simulink model "GMCLIB_Clark_BAM_FLT"  (Simulink 7.3)
settings: Solver=ode45  StartTime=0.0  StopTime=10.0  RelTol=1e-3
settings Model: Creator=B17364  LastModifiedBy=B17364

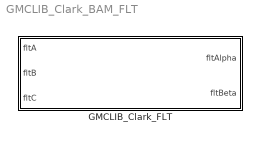
== system GMCLIB_Clark_BAM_FLT ==
  GMCLIB_Clark_FLT : Subsystem  mask(GMCLIB_Clark_FLT){}
      mask help: Bit accurate model of Clarke transformation 3ph -> 2ph.
      mask init:
      | pos = get_param(gcb, 'Position');width = pos(3) - pos(1); height = pos(4) - pos(2);tX=width/2;tY=height*0.9;
      mask Display: color('black');port_label('input',1,'fltA');port_label('input',2,'fltB');port_label('input',3,'fltC');port_label('output',1,'fltAlpha');port_label('output',2,'fltBeta');color('black');disp('GMCLIB_Clark_FLT');color('blue');text(tX,tY, 'BAM', 'horizontalAlignment', 'center');

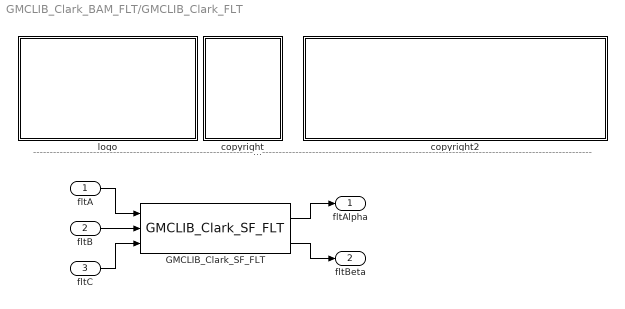
== system GMCLIB_Clark_BAM_FLT/GMCLIB_Clark_FLT ==
  note: ---------------------------------------------------------------------------------------------------------------------------------------------------------------------------------------------------
  fltA : Inport  OutDataType=fixdt(1, 16)  OutScaling=2^0
  fltB : Inport  Port=2  OutDataType=fixdt(1, 16)  OutScaling=2^0
  fltC : Inport  Port=3  OutDataType=fixdt(1, 16)  OutScaling=2^0
  GMCLIB_Clark_SF_FLT : S-Function  FunctionName=GMCLIB_Clark_SF_FLT  EnableBusSupport=off
  copyright : Subsystem
      mask Display: text(10,90,'FILE:');text(10,75,'DESRIPTION:')text(10,60,'COPYRIGHT:')text(10,45,'VERSION:')text(10,30,'DATE:')
  copyright2 : Subsystem
      mask Display: text(10,90,'GMCLIB_Clark_BAM_FLT.mdl');text(10,75,'Clarke transformation.');text(10,60,'Freescale')text(10,45,'0.1');text(10,30,'29-Aug-2011');
  logo : Subsystem
      mask Display: image(imread('logo.jpg'))
  fltAlpha : Outport  OutDataType=fixdt(1, 16)  OutScaling=2^0
  fltBeta : Outport  Port=2  OutDataType=fixdt(1, 16)  OutScaling=2^0
  wires:
  fltA/1 -> GMCLIB_Clark_SF_FLT/1
  fltB/1 -> GMCLIB_Clark_SF_FLT/2
  fltC/1 -> GMCLIB_Clark_SF_FLT/3
  GMCLIB_Clark_SF_FLT/1 -> fltAlpha/1
  GMCLIB_Clark_SF_FLT/2 -> fltBeta/1

== system GMCLIB_Clark_BAM_FLT/GMCLIB_Clark_FLT/copyright ==

== system GMCLIB_Clark_BAM_FLT/GMCLIB_Clark_FLT/copyright2 ==

== system GMCLIB_Clark_BAM_FLT/GMCLIB_Clark_FLT/logo ==
